simulink model "OC4_Kalman_Filter"  (R2023b)
settings: Solver=ode4  StartTime=0.0  StopTime=TMax  FixedStep=DT  MaxStep=DT  RelTol=1e-3  EnableMultiTasking=on
undefined symbols (not defined in the file): Ared, Bred, DHred, DiscIntNeverNeededParam, Discrete, Hred, Ki, Klqg, Max_pitch, Max_pitch_rate, Min_pitch, Min_pitch_rate, Qkf, Ref, Rkf, Time, y_OP
libraries: ctrlSharedLib x1
settings Model: Creator=bjonkman  LastModifiedBy=ianam
settings SolverCC: AlgebraicLoopSolver=TrustRegion
settings DataIOCC: LimitDataPoints=on  SaveFormat=Array  SignalLoggingSaveFormat=ModelDataLogs  SaveOutput=off  SaveTime=off  ReturnWorkspaceOutputs=off  SignalLoggingName=sigsOut
settings OptimizationCC: ExpressionDepthLimit=2147483647  LifeSpan=inf
settings DebuggingCC: SaveWithParameterizedLinksMsg=none  UnderspecifiedInitializationDetection=Classic  MergeDetectMultiDrivingBlocksExec=none  SignalResolutionControl=TryResolveAllWithWarning  MultiTaskDSMMsg=warning  MultiTaskCondExecSysMsg=none  FcnCallInpInsideContextMsg=warning  UnconnectedInputMsg=warning  UnconnectedOutputMsg=warning  UnconnectedLineMsg=warning  StateNameClashWarn=warning  SFUnexpectedBacktrackingDiag=warning  SFNoUnconditionalDefaultTransitionDiag=warning  SFExecutionAtInitializationDiag=none  ArithmeticOperatorsInVariantConditions=warning
settings HardwareCC: ProdBitPerPointer=32  ProdBitPerSizeT=32  ProdBitPerPtrDiffT=32  ProdLargestAtomicFloat=None  ProdIntDivRoundTo=Undefined  ProdEndianess=Unspecified  ProdWordSize=32  ProdHWDeviceType=32-bit Generic  TargetUnknown=on
settings ModelReferenceCC: EnableRefExpFcnMdlSchedulingChecks=on  PropagateSignalLabelsOutOfModel=off
settings SFSimCC: SimUseLocalCustomCode=off  CustomCodeUndefinedFunction=UseInterfaceOnly
settings RTWCC: RTWUseLocalCustomCode=off  DLArmComputeVersion=19.05
settings CodeAppCC: StateflowObjectComments=on
settings GRTTargetCC: TargetLangStandard=C89/C90 (ANSI)  CombineOutputUpdateFcns=off  GRTInterface=on
settings ConfigComp: CovMetricSettings=dw  CovSaveCumulativeToWorkspaceVar=on  CovSaveSingleToWorkspaceVar=on  CovExternalEMLEnable=off

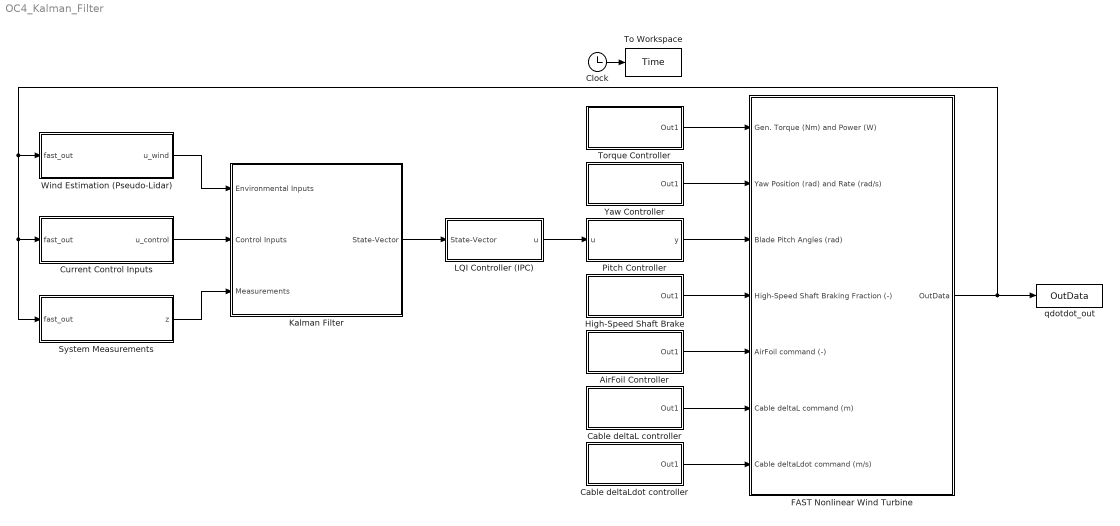
== system OC4_Kalman_Filter ==
  AirFoil Controller : Subsystem
  Cable deltaL controller : Subsystem
  Cable deltaLdot controller : Subsystem
  Clock : Clock
  Current Control Inputs : MATLAB Function  TreatAsAtomicUnit=on
  FAST Nonlinear Wind Turbine : Subsystem  mask(FAST Nonlinear Wind Turbine){}
      mask help: This block contains the FAST S-Function.
      mask init:
      | clear FAST_SFunc
  High-Speed Shaft Brake : Subsystem
  Kalman Filter : Subsystem
  LQI Controller (IPC) : Subsystem
  Pitch Controller : Subsystem
  System Measurements : MATLAB Function  TreatAsAtomicUnit=on
  To Workspace : ToWorkspace  VariableName=Time  SampleTime=-1
  Torque Controller : Subsystem
  Wind Estimation (Pseudo-Lidar) : MATLAB Function  TreatAsAtomicUnit=on
  Yaw Controller : Subsystem
  qdotdot_out : ToWorkspace  VariableName=OutData  SampleTime=-1
  wires:
  Clock/1 -> To Workspace/1
  FAST Nonlinear Wind Turbine/1(OutData) -> System Measurements/1(fast_out), Current Control Inputs/1(fast_out), Wind Estimation (Pseudo-Lidar)/1(fast_out), qdotdot_out/1
  Torque Controller/1(Out1) -> FAST Nonlinear Wind Turbine/1(Gen. Torque (Nm) and Power (W))
  Yaw Controller/1(Out1) -> FAST Nonlinear Wind Turbine/2(Yaw Position (rad) and Rate (rad/s))
  Pitch Controller/1(y) -> FAST Nonlinear Wind Turbine/3(Blade Pitch Angles (rad))
  High-Speed Shaft Brake/1(Out1) -> FAST Nonlinear Wind Turbine/4(High-Speed Shaft Braking Fraction (-))
  AirFoil Controller/1(Out1) -> FAST Nonlinear Wind Turbine/5(AirFoil command (-))
  Cable deltaL controller/1(Out1) -> FAST Nonlinear Wind Turbine/6(Cable deltaL command (m))
  Cable deltaLdot controller/1(Out1) -> FAST Nonlinear Wind Turbine/7(Cable deltaLdot command (m/s))
  LQI Controller (IPC)/1(u) -> Pitch Controller/1(u)
  Wind Estimation (Pseudo-Lidar)/1(u_wind) -> Kalman Filter/1(Environmental Inputs)
  Current Control Inputs/1(u_control) -> Kalman Filter/2(Control Inputs)
  System Measurements/1(z) -> Kalman Filter/3(Measurements)
  Kalman Filter/1(State-Vector) -> LQI Controller (IPC)/1(State-Vector)

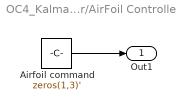
== system OC4_Kalman_Filter/AirFoil Controller ==
  Airfoil command : Constant  Value=zeros(1,3)'
  Out1 : Outport
  wires:
  Airfoil command/1 -> Out1/1

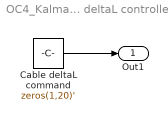
== system OC4_Kalman_Filter/Cable deltaL controller ==
  Cable deltaL command : Constant  Value=zeros(1,20)'
  Out1 : Outport
  wires:
  Cable deltaL command/1 -> Out1/1

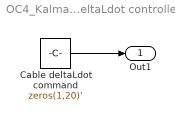
== system OC4_Kalman_Filter/Cable deltaLdot controller ==
  Cable deltaLdot command : Constant  Value=zeros(1,20)'
  Out1 : Outport
  wires:
  Cable deltaLdot command/1 -> Out1/1

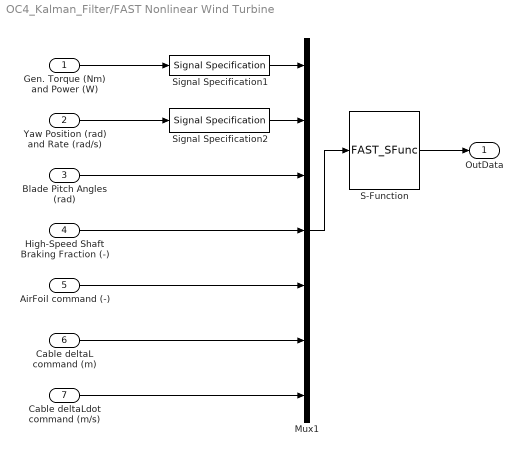
== system OC4_Kalman_Filter/FAST Nonlinear Wind Turbine ==
  Gen. Torque (Nm) and Power (W) : Inport
  Yaw Position (rad) and Rate (rad/s) : Inport  Port=2
  Blade Pitch Angles (rad) : Inport  Port=3
  High-Speed Shaft Braking Fraction (-) : Inport  Port=4
  AirFoil command (-) : Inport  Port=5
  Cable deltaL command (m) : Inport  Port=6
  Cable deltaLdot command (m/s) : Inport  Port=7
  Mux1 : Mux  Inputs=7
  S-Function : S-Function  FunctionName=FAST_SFunc  Parameters=FAST_InputFileName, TMax, 0  SFunctionDeploymentMode=off  EnableBusSupport=off
  Signal Specification1 : SignalSpecification  OutDataTypeStr=double  Dimensions=2
  Signal Specification2 : SignalSpecification  OutDataTypeStr=double  Dimensions=2
  OutData : Outport
  wires:
  Gen. Torque (Nm) and Power (W)/1 -> Signal Specification1/1
  S-Function/1 -> OutData/1
  Mux1/1 -> S-Function/1
  Blade Pitch Angles (rad)/1 -> Mux1/3
  Yaw Position (rad) and Rate (rad/s)/1 -> Signal Specification2/1
  Signal Specification1/1 -> Mux1/1
  Signal Specification2/1 -> Mux1/2
  High-Speed Shaft Braking Fraction (-)/1 -> Mux1/4
  AirFoil command (-)/1 -> Mux1/5
  Cable deltaL command (m)/1 -> Mux1/6
  Cable deltaLdot command (m/s)/1 -> Mux1/7

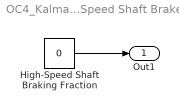
== system OC4_Kalman_Filter/High-Speed Shaft Brake ==
  High-Speed Shaft Braking Fraction : Constant  Value=0
  Out1 : Outport
  wires:
  High-Speed Shaft Braking Fraction/1 -> Out1/1

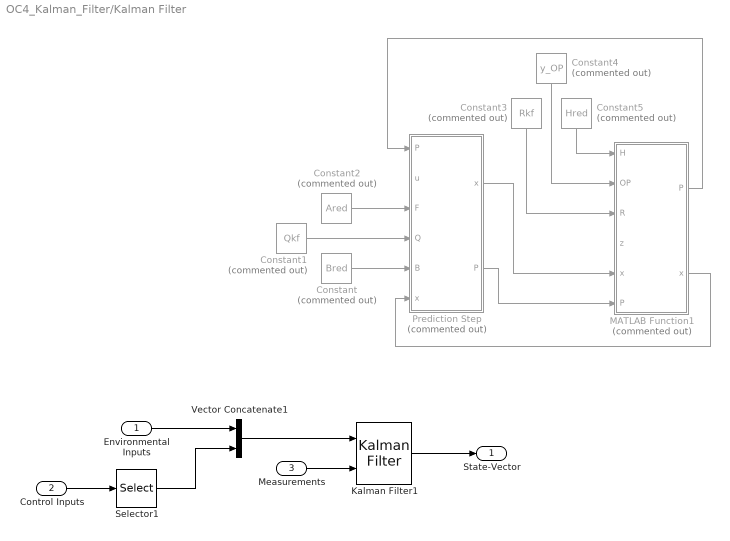
== system OC4_Kalman_Filter/Kalman Filter ==
  Environmental Inputs : Inport
  Control Inputs : Inport  Port=2
  Measurements : Inport  Port=3
  Constant : Constant  Commented=on  Value=Bred
  Constant1 : Constant  Commented=on  Value=Qkf
  Constant2 : Constant  Commented=on  Value=Ared
  Constant3 : Constant  Commented=on  Value=Rkf
  Constant4 : Constant  Commented=on  Value=y_OP
  Constant5 : Constant  Commented=on  Value=Hred
  Kalman Filter1 : ctrlSharedLib/Kalman Filter  TimeDomain=Discrete-Time  UseCurrentEstimator=on  ModelSource=Individual A, B, C, D matrices  ModelSourceVariable=ss(0.95,1,1,0,1)  A=Ared  B=Bred  C=Hred  D=DHred  NumberOfStates=1  NumberOfInputs=1  NumberOfOutputs=1  InitialEstimateSource=Dialog  X0=zeros(size(Ared,1),1)  P0=10  UseK=off  UseGH=off  NumberOfProcessNoiseInputs=1  G=1  TimeInvariantG=on  H=0  TimeInvariantH=on  Q=Qkf  TimeInvariantQ=on  R=Rkf  TimeInvariantR=on  N=0  TimeInvariantN=on  AddInputPort=on  AddEnablePort=off  OutputEstimatedY=off  OutputP=off  Ts=-1
  MATLAB Function1 : MATLAB Function  Commented=on  TreatAsAtomicUnit=on
  Prediction Step : MATLAB Function  Commented=on  TreatAsAtomicUnit=on
  Selector1 : Selector  InputPortWidth=5  IndexOptions=Index vector (dialog)  Indices=[5,4]  OutputSizes=1
  Vector Concatenate1 : Concatenate
  State-Vector : Outport
  wires:
  MATLAB Function1/2(x) -> Prediction Step/6("x ")
  MATLAB Function1/1(P) -> Prediction Step/1("P ")
  Prediction Step/1(x) -> MATLAB Function1/5("x ")
  Prediction Step/2(P) -> MATLAB Function1/6("P ")
  Constant5/1 -> MATLAB Function1/1(H)
  Constant1/1 -> Prediction Step/4(Q)
  Constant4/1 -> MATLAB Function1/2(OP)
  Constant2/1 -> Prediction Step/3(F)
  Constant3/1 -> MATLAB Function1/3(R)
  Constant/1 -> Prediction Step/5(B)
  Selector1/1 -> Vector Concatenate1/2
  Environmental Inputs/1 -> Vector Concatenate1/1
  Control Inputs/1 -> Selector1/1
  Vector Concatenate1/1 -> Kalman Filter1/1
  Measurements/1 -> Kalman Filter1/2
  Kalman Filter1/1 -> State-Vector/1

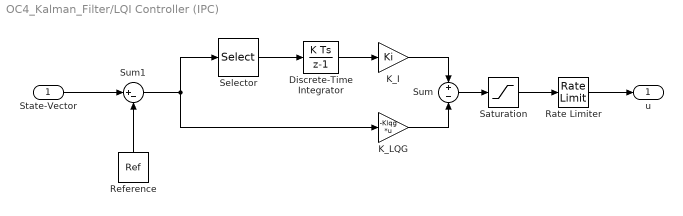
== system OC4_Kalman_Filter/LQI Controller (IPC) ==
  State-Vector : Inport
  Discrete-Time Integrator : DiscreteIntegrator  SampleTime=-1  ICPrevOutput=DiscIntNeverNeededParam  ICPrevScaledInput=DiscIntNeverNeededParam
  K_I : Gain  Gain=Ki
  K_LQG : Gain  Gain=-Klqg  Multiplication=Matrix(K*u)
  Rate Limiter : RateLimiter  RisingSlewLimit=Max_pitch_rate  FallingSlewLimit=Min_pitch_rate  SampleTimeMode=inherited
  Reference : Constant  Value=Ref
  Saturation : Saturate  UpperLimit=Max_pitch  LowerLimit=Min_pitch
  Selector : Selector  InputPortWidth=13  IndexOptions=Index vector (dialog)  Indices=[10]  OutputSizes=1
  Sum : Sum  Inputs=+|-
  Sum1 : Sum  Inputs=|+-
  u : Outport
  wires:
  Sum1/1 -> K_LQG/1, Selector/1
  K_LQG/1 -> Sum/2
  K_I/1 -> Sum/1
  Sum/1 -> Saturation/1
  Saturation/1 -> Rate Limiter/1
  Rate Limiter/1 -> u/1
  Selector/1 -> Discrete-Time Integrator/1
  Discrete-Time Integrator/1 -> K_I/1
  State-Vector/1 -> Sum1/1
  Reference/1 -> Sum1/2

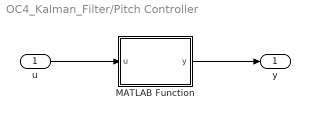
== system OC4_Kalman_Filter/Pitch Controller ==
  u : Inport
  MATLAB Function : MATLAB Function  TreatAsAtomicUnit=on
  y : Outport
  wires:
  u/1 -> MATLAB Function/1(u)
  MATLAB Function/1(y) -> y/1

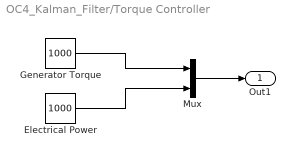
== system OC4_Kalman_Filter/Torque Controller ==
  Electrical Power : Constant  Value=1000
  Generator Torque : Constant  Value=1000
  Mux : Mux  Inputs=2
  Out1 : Outport
  wires:
  Mux/1 -> Out1/1
  Generator Torque/1 -> Mux/1
  Electrical Power/1 -> Mux/2

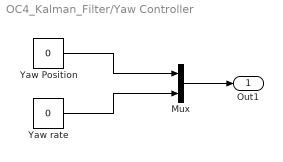
== system OC4_Kalman_Filter/Yaw Controller ==
  Mux : Mux  Inputs=2
  Yaw Position : Constant  Value=0
  Yaw rate : Constant  Value=0
  Out1 : Outport
  wires:
  Mux/1 -> Out1/1
  Yaw Position/1 -> Mux/1
  Yaw rate/1 -> Mux/2

== matlab function OC4_Kalman_Filter/System Measurements ==
  data: fast_out input; z output
function z = getMeasurements(fast_out)

%% Extract "Measurements" from FAST Output Vector
PtfmPitch = fast_out(24); % degrees
PtfmRoll  = fast_out(23); % degrees
RotSpeed  = fast_out(6); % RPM

z = [PtfmPitch;
     RotSpeed];

== matlab function OC4_Kalman_Filter/Pitch Controller/MATLAB Function ==
  data: u input; y output size=3
function y = fcn(u)

% Extract blade pitch
%current_pitch = u(11);

% Define new blade pitch
%if current_pitch == 0
%    blade_pitch = 14;
%else
%    adjust = rand;
%    blade_pitch = 14 + 0.2*(adjust - 0.5);
%end
%
% % Convert degrees to rads
%blade_pitch = blade_pitch*(pi/180);

% % Output blade pitch
%y = [blade_pitch;
%     blade_pitch;
%     blade_pitch];

y = [u,u,u]';

== matlab function OC4_Kalman_Filter/Kalman Filter/Prediction Step ==
  data: P input; u input; F input; Q input; B input; x input; x output; P output
function [x,P] = predict(P,u,F,Q,B,x)

% Update state vector
x = F*x + B*u;

% Update process covariance
P = F*P*F' + Q;

== matlab function OC4_Kalman_Filter/Current Control Inputs ==
  data: fast_out input; u_control output
function u_control = getControl(fast_out)

% Extract blade pitch commands from FAST
blade_pitch_1 = fast_out(11);
blade_pitch_2 = fast_out(12);
blade_pitch_3 = fast_out(13);
blade_pitch_C = mean([blade_pitch_1,blade_pitch_2,blade_pitch_3]);

% Extract generator torque command from FAST
gen_torque = fast_out(57);

u_control = [blade_pitch_1;
             blade_pitch_2;
             blade_pitch_3;
             blade_pitch_C;
             gen_torque];

== matlab function OC4_Kalman_Filter/Wind Estimation (Pseudo-Lidar) ==
  data: fast_out input; u_wind output
function u_wind = getWind(fast_out)

% Extract wind from FAST
wind = fast_out(2);

% Add noise to wind to simulate lidar accuracy
% ...

% Output wind velocity
u_wind = wind;

== matlab function OC4_Kalman_Filter/Kalman Filter/MATLAB Function1 ==
  data: P output; H input; OP input; R input; z input; x input; x output; P input
function [P,x] = update(H,OP,R,z,x,P)
   
P = P + zeros(size(F));
x = x + zeros(size(F,1),1);

S = H*P*H' + R; % Project system uncertainty into measurement space & add measurement uncertainty
K = P*H'*inv(S);
y = z-(H*x + OP); % Error term
x = x+K*y;
KH = K*H;
P = (eye(size(KH))-KH)*P;
